simulink model "lineAndEdgeDetection"  (R2018a)
settings: Solver=FixedStepAuto  StartTime=0.0  StopTime=10.0  FixedStep=0.1  RelTol=1e-3
model workspace (MAT data in the model file):
  clusterProximityThreshold = 0.05
  lineTrackingThreshold = 0.2
  netAngleThreshold = 0.314159265359
  scalerho = 0.002
undefined symbols (not defined in the file or in its folder): gray
libraries: visiontextngfix x3, visiontransforms x3, dspindex x2, visionanalysis x1, visionstatistics x1, visiongeotforms x1
settings Model: Creator=vuwij  LastModifiedBy=vuwij
settings DataIOCC: SaveOutput=off  SaveTime=off
settings OptimizationCC: EnhancedBackFolding=on  PassReuseOutputArgsAs=Individual arguments  MaxStackSize=64  OptimizeBlockOrder=speed  DifferentSizesBufferReuse=on  OptimizationCustomize=off
settings DebuggingCC: ParameterTunabilityLossMsg=error
settings HardwareCC: ProdBitPerPointer=32  ProdBitPerSizeT=32  ProdBitPerPtrDiffT=32  ProdLargestAtomicFloat=None  ProdIntDivRoundTo=Undefined  ProdEndianess=Unspecified  ProdWordSize=32  ProdHWDeviceType=Generic->Unspecified (assume 32-bit Generic)
settings SFSimCC: MATLABDynamicMemAlloc=off
settings RTWCC: SystemTargetFile=ert.tlc  HardwareBoard=Robot Operating System (ROS)  TLCOptions="-aInlineSetEventsForThisBaseRateFcn=TLC_FALSE -aSuppressMultiTaskScheduler=TLC_FALSE  -aRateBasedStepFcn=0"  TemplateMakefile=ert_default_tmf  GenerateReport=on  Toolchain=Catkin  IncludeHyperlinkInReport=on  LaunchReport=on  TargetLang=C++  GenerateTraceInfo=on  GenerateTraceReport=on  GenerateTraceReportSl=on  GenerateTraceReportSf=on  GenerateTraceReportEml=on
settings CodeAppCC: ForceParamTrailComments=on  IgnoreCustomStorageClasses=off  OperatorAnnotations=on  SimulinkDataObjDesc=on  SFDataObjDesc=on  InsertBlockDesc=on
settings ERTTargetCC: SupportVariableSizeSignals=on

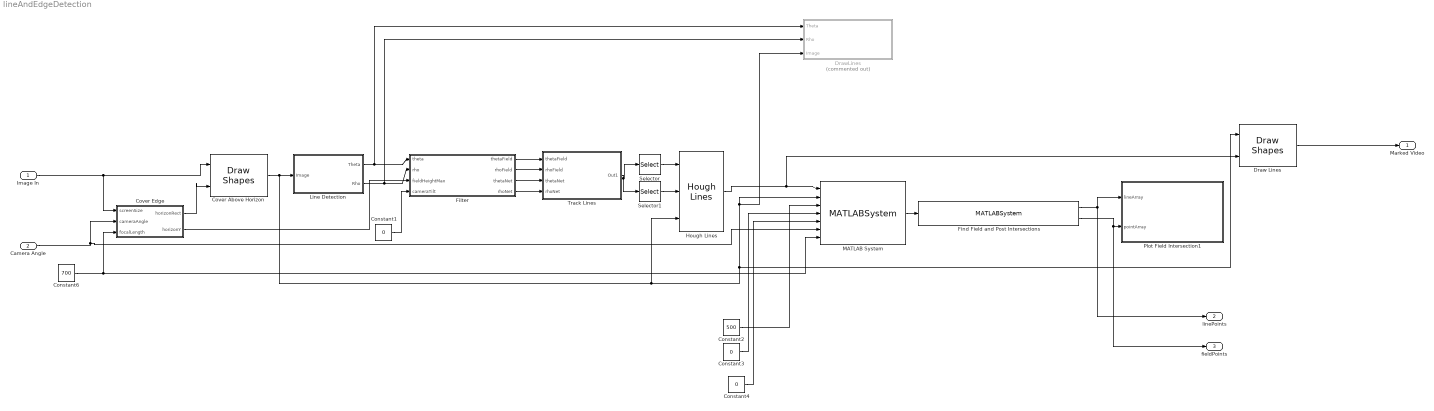
== system lineAndEdgeDetection ==
  Image In : Inport  OutDataTypeStr=uint8  PortDimensions=[480 640]  SampleTime=[0.1,0]
  Camera Angle : Inport  Port=2  PortDimensions=1
  Constant1 : Constant  Value=0
  Constant2 : Constant  Value=500
  Constant3 : Constant  Value=0
  Constant4 : Constant  Value=0
  Constant6 : Constant  Value=700
  Cover Above Horizon : visiontextngfix/Draw Shapes  shape=Rectangles  fill=on  lineWidth=1  fillClrSource=Specify via dialog  display=Black  intensity=200  color=[255 0 0]  opacity=0.8  viewport=Entire image  antialiasing=off  inType=Obsolete  imagePorts=One multidimensional signal  prodOutputMode=Binary point scaling  prodOutputWordLength=32  prodOutputFracLength=14  memoryMode=Specify word length  memoryWordLength=16  memoryFracLength=14  roundingMode=Floor  overflowMode=off
      settings: SourceProductName=Computer Vision System Toolbox
  Cover Edge : MATLAB Function  TreatAsAtomicUnit=on
  Draw Lines : visiontextngfix/Draw Shapes  shape=Lines  fill=off  lineWidth=1  fillClrSource=Specify via dialog  display=White  intensity=200  color=[255 0 0]  opacity=0.6  viewport=Entire image  antialiasing=on  inType=Obsolete  imagePorts=One multidimensional signal  prodOutputMode=Binary point scaling  prodOutputWordLength=32  prodOutputFracLength=14  memoryMode=Specify word length  memoryWordLength=16  memoryFracLength=14  roundingMode=Floor  overflowMode=off
      settings: SourceProductName=Computer Vision System Toolbox
  DrawLines : Subsystem  Commented=on
  Filter : MATLAB Function  TreatAsAtomicUnit=on
  Find Field and Post Intersections : MATLABSystem  System=findFieldAndPostIntersections  SimulateUsing=Interpreted execution
      mask Type: findFieldAndPostIntersections
      mask Display:
      | disp('findFieldAndPostIntersections');
      | port_label('input',1,'lineArray');
      | port_label('output',1,'lineArray');
      | port_label('output',2,'pointArray');
  Hough Lines : visiontransforms/Hough Lines  sineCompMethod=Trigonometric function  thetaRes=pi/180  firstCoeffMode=Specify word length  firstCoeffWordLength=16  firstCoeffFracLength=15  prodOutputMode=Binary point scaling  prodOutputWordLength=32  prodOutputFracLength=16  roundingMode=Nearest  overflowMode=on
      settings: SourceProductName=Computer Vision System Toolbox  SourceProductBaseCode=VP
  Line Detection : Subsystem
  MATLAB System : MATLABSystem  System=map2Dto3D  SimulateUsing=Interpreted execution
      mask Type: map2Dto3D
      mask Display:
      | disp('map2Dto3D');
      | port_label('input',1,'lines');
      | port_label('input',2,'img');
      | port_label('input',3,'robotHeight');
      | port_label('input',4,'d');
      | port_label('input',5,'robotAngle');
      | port_label('input',6,'cameraAngle');
      | port_label('input',7,'focalLength');
      | port_label('output',1,'lines3D');
  Plot Field Intersection1 : MATLAB Function  TreatAsAtomicUnit=on
  Selector : Selector  NumberOfDimensions=2  InputPortWidth=3  IndexOptions=Select all,Index vector (dialog)  Indices=[1 3],1  OutputSizes=1,1
  Selector1 : Selector  NumberOfDimensions=2  InputPortWidth=3  IndexOptions=Select all,Index vector (dialog)  Indices=[1 3],2  OutputSizes=1,1
  Track Lines : Subsystem
  Marked Video : Outport  OutDataTypeStr=uint8  SampleTime=[0,1]
  linePoints : Outport  Port=2  OutDataTypeStr=double  SampleTime=[0,1]
  fieldPoints : Outport  Port=3  OutDataTypeStr=double  SampleTime=[0,1]
  wires:
  Line Detection/1(Theta) -> Filter/1(theta), DrawLines/1(Theta)
  Line Detection/2(Rho) -> Filter/2(rho), DrawLines/2(Rho)
  Constant1/1 -> Filter/4(cameraTilt)
  Filter/2(rhoField) -> Track Lines/2("rhoField ")
  Filter/3(thetaNet) -> Track Lines/3(thetaNet)
  Filter/4(rhoNet) -> Track Lines/4(rhoNet)
  Hough Lines/1 -> MATLAB System/1, Draw Lines/2
  Constant2/1 -> MATLAB System/3
  Constant3/1 -> MATLAB System/4
  Constant4/1 -> MATLAB System/5
  Constant6/1 -> Cover Edge/3(focalLength), MATLAB System/7
  Track Lines/1(Out1) -> Selector/1, Selector1/1
  Selector/1 -> Hough Lines/1
  Selector1/1 -> Hough Lines/2
  Draw Lines/1 -> Marked Video/1
  Cover Above Horizon/1 -> Draw Lines/1, DrawLines/3(Image), MATLAB System/2, Hough Lines/3, Line Detection/1(Image)
  Camera Angle/1 -> Cover Edge/2(cameraAngle), MATLAB System/6
  Cover Edge/1(horizonRect) -> Cover Above Horizon/2
  Filter/1(thetaField) -> Track Lines/1(thetaField)
  Cover Edge/2(horizonY) -> Filter/3(fieldHeightMax)
  Find Field and Post Intersections/2 -> fieldPoints/1, Plot Field Intersection1/2(pointArray)
  MATLAB System/1 -> Find Field and Post Intersections/1
  Image In/1 -> Cover Edge/1(screenSize), Cover Above Horizon/1
  Find Field and Post Intersections/1 -> linePoints/1, Plot Field Intersection1/1(lineArray)

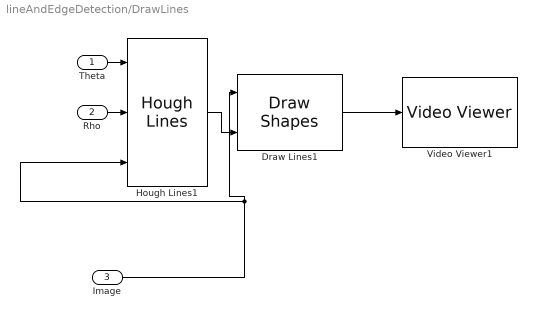
== system lineAndEdgeDetection/DrawLines ==
  Theta : Inport
  Rho : Inport  Port=2
  Image : Inport  Port=3
  Draw Lines1 : visiontextngfix/Draw Shapes  shape=Lines  fill=off  lineWidth=1  fillClrSource=Specify via dialog  display=White  intensity=200  color=[255 0 0]  opacity=0.6  viewport=Entire image  antialiasing=off  inType=Obsolete  imagePorts=One multidimensional signal  prodOutputMode=Binary point scaling  prodOutputWordLength=32  prodOutputFracLength=14  memoryMode=Specify word length  memoryWordLength=16  memoryFracLength=14  roundingMode=Floor  overflowMode=off
      settings: SourceProductName=Computer Vision System Toolbox
  Hough Lines1 : visiontransforms/Hough Lines  sineCompMethod=Trigonometric function  thetaRes=pi/180  firstCoeffMode=Specify word length  firstCoeffWordLength=16  firstCoeffFracLength=15  prodOutputMode=Binary point scaling  prodOutputWordLength=32  prodOutputFracLength=16  roundingMode=Nearest  overflowMode=on
      settings: SourceProductName=Computer Vision System Toolbox  SourceProductBaseCode=VP
  Video Viewer1 : VideoViewer  colormapValue=gray(256)  FigPos=[-205.666666666667 996 1136 624]
  wires:
  Theta/1 -> Hough Lines1/1
  Draw Lines1/1 -> Video Viewer1/1
  Hough Lines1/1 -> Draw Lines1/2
  Image/1 -> Hough Lines1/3, Draw Lines1/1
  Rho/1 -> Hough Lines1/2

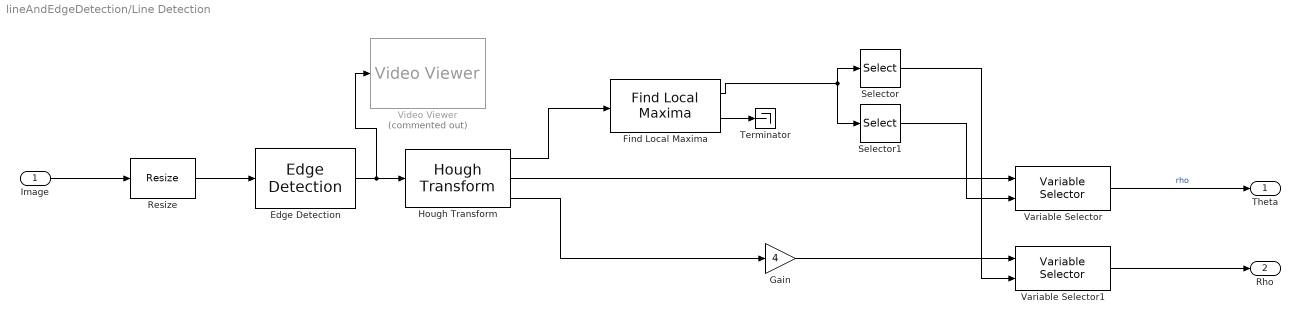
== system lineAndEdgeDetection/Line Detection ==
  Image : Inport
  Edge Detection : visionanalysis/Edge Detection  method=Prewitt  outputType=Binary image  userDefinedThreshold=off  thresholdSource=Input port  threshold=20  thresholdTuning=6  edgeThinning=on  threshold_canny=[0.25 0.60]  autoPercent=70  sigma=1  roundingMode=Floor  overflowMode=off  prodOutputMode=Binary point scaling  prodOutputWordLength=32  prodOutputFracLength=8  prodOutputSlope=2^-8  accumSlope=2^-8  outputSlope=2^-4
      settings: SourceProductName=Computer Vision System Toolbox  SourceProductBaseCode=VP
  Find Local Maxima : visionstatistics/Find Local Maxima  num_peaks=20  nhood_size=[201 51]  src_thresh=Obsolete9b  src_thresh_inuse=Specify via dialog  threshold=27  inputIsHough=on  dt_peak=uint32  isOutVarDim=off  dt_count=uint32
      settings: SourceProductName=Computer Vision System Toolbox  SourceProductBaseCode=VP
  Gain : Gain  Gain=4
  Hough Transform : visiontransforms/Hough Transform  theta_res=pi/180  rho_res=1  out_theta_rho=on  outdtmode=double  firstCoeffMode=Binary point scaling  firstCoeffWordLength=16  firstCoeffFracLength=14  secondCoeffMode=Binary point scaling  secondCoeffWordLength=32  secondCoeffFracLength=16  outputMode=Binary point scaling  outputWordLength=16  outputFracLength=0  accumMode=Binary point scaling  accumWordLength=32  accumFracLength=20  prodOutputMode=Binary point scaling  prodOutputWordLength=32  prodOutputFracLength=20  memoryMode=Binary point scaling  memoryWordLength=32  memoryFracLength=16  roundingMode=Nearest  overflowMode=on
      settings: SourceProductName=Computer Vision System Toolbox  SourceProductBaseCode=VP
  Resize : visiongeotforms/Resize  specify=Output size as a percentage of input size  rfactor=[25 25]  outCols=25  outRows=25  outRowsCols=[25 35]  interp_method=Bilinear  antialias=off  useROI=off  roiFlag=off  prodOutputMode=Binary point scaling  prodOutputWordLength=32  prodOutputFracLength=10  roundingMode=Nearest  overflowMode=on
      settings: SourceProductName=Computer Vision System Toolbox  SourceProductBaseCode=VP
  Selector : Selector  NumberOfDimensions=2  InputPortWidth=2  IndexOptions=Select all,Index vector (dialog)  Indices=1,2  OutputSizes=1,1
  Selector1 : Selector  NumberOfDimensions=2  InputPortWidth=2  IndexOptions=Select all,Index vector (dialog)  Indices=0,1  OutputSizes=1,1
  Terminator : Terminator
  Variable Selector : dspindex/Variable Selector  NumInputs=1  rowsOrCols=Columns  IdxMode=Variable  Elements=[1 3]  ZerOneIdxMode=One-based  errmode=Clip Index  FillMode=on  FillValues=0
  Variable Selector1 : dspindex/Variable Selector  NumInputs=1  rowsOrCols=Columns  IdxMode=Variable  Elements=[1 3]  ZerOneIdxMode=One-based  errmode=Clip Index  FillMode=on  FillValues=0
  Video Viewer : VideoViewer  Commented=on  FigPos=[727 756 635 435]
  Theta : Outport
  Rho : Outport  Port=2
  wires:
  Image/1 -> Resize/1
  Gain/1 -> Variable Selector1/1
  Resize/1 -> Edge Detection/1
  Edge Detection/1 -> Hough Transform/1, Video Viewer/1
  Variable Selector1/1 -> Rho/1
  Variable Selector/1 -> Theta/1  "rho"
  Hough Transform/3 -> Gain/1
  Selector1/1 -> Variable Selector/2
  Selector/1 -> Variable Selector1/2
  Find Local Maxima/1 -> Selector/1, Selector1/1
  Hough Transform/2 -> Variable Selector/1
  Hough Transform/1 -> Find Local Maxima/1
  Find Local Maxima/2 -> Terminator/1

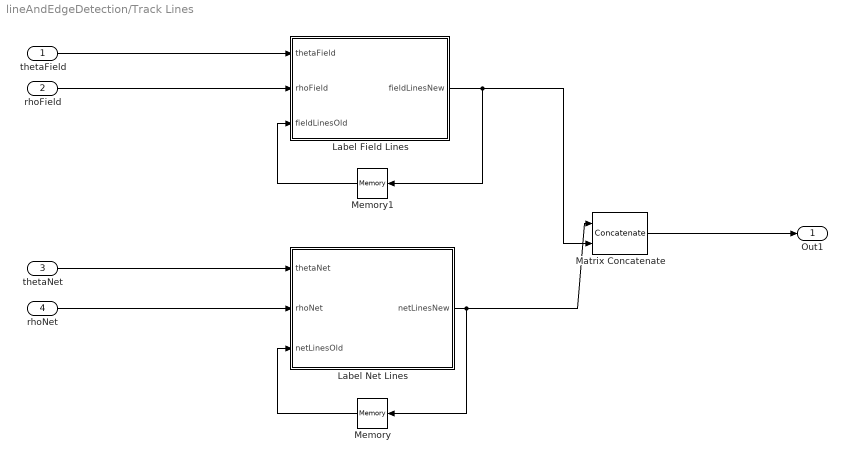
== system lineAndEdgeDetection/Track Lines ==
  thetaField : Inport
  "rhoField " : Inport  Port=2
  thetaNet : Inport  Port=3
  rhoNet : Inport  Port=4
  Label Field Lines : MATLAB Function  TreatAsAtomicUnit=on
  Label Net Lines : MATLAB Function  TreatAsAtomicUnit=on
  Matrix Concatenate : Concatenate  Mode=Multidimensional array
  Memory : Memory  InitialCondition=[0,0;0,0;0,0;0,0]
  Memory1 : Memory  InitialCondition=[0,0;0,0;0,0;0,0;0,0]
  Out1 : Outport
  wires:
  Matrix Concatenate/1 -> Out1/1
  Label Field Lines/1(fieldLinesNew) -> Memory1/1, Matrix Concatenate/2
  Memory1/1 -> Label Field Lines/3(fieldLinesOld)
  thetaField/1 -> Label Field Lines/1(thetaField)
  "rhoField "/1 -> Label Field Lines/2(rhoField)
  Memory/1 -> Label Net Lines/3(netLinesOld)
  Label Net Lines/1(netLinesNew) -> Memory/1, Matrix Concatenate/1
  rhoNet/1 -> Label Net Lines/2(rhoNet)
  thetaNet/1 -> Label Net Lines/1(thetaNet)

== matlab function lineAndEdgeDetection/Cover Edge ==
  data: horizonRect output; horizonY output; screenSize input; cameraAngle input; focalLength input
function [horizonRect, horizonY] = fcn(screenSize, cameraAngle, focalLength)
    [l, w] = size(screenSize);
    
    horizonY = l/2 - tan(cameraAngle) * focalLength;
    horizonRect = uint32([0, 0, w, horizonY]);

== matlab function lineAndEdgeDetection/Track Lines/Label Net Lines ==
  data: thetaNet input; netLinesNew output; rhoNet input; netLinesOld input; lineTrackingThreshold parameter; scalerho parameter
function netLinesNew = labelNetLines(thetaNet, rhoNet, netLinesOld, lineTrackingThreshold, scalerho)
    % Keep the memory of the new lines
    netLinesNew = zeros(4,2);
    if any(netLinesOld)
        netLinesNew = netLinesOld;
    end
    
    % Update if anything changed
    totalLineCount = 0;
    for i = 1:6
       if (thetaNet(i) == 0 && rhoNet(i) == 0)
           continue;
       else
           totalLineCount = totalLineCount + 1;
       end
    end
    
    if (totalLineCount == 2)
        if(rhoNet(2) < rhoNet(1))
            netLinesNew(1,1) = thetaNet(1);
            netLinesNew(1,2) = rhoNet(1);
            netLinesNew(2,1) = thetaNet(2);
            netLinesNew(2,2) = rhoNet(2);
        else
            netLinesNew(1,1) = thetaNet(2);
            netLinesNew(1,2) = rhoNet(2);
            netLinesNew(2,1) = thetaNet(1);
            netLinesNew(2,2) = rhoNet(1);
        end
    end
    
    if (totalLineCount == 1)
        if(netLinesNew(1,1) ~= 0 && netLinesNew(2,1) ~= 0 && netLinesNew(1,2) ~= 0 && netLinesNew(2,2) ~= 0) % Seen both lines already
            theta1 = netLinesNew(1,1);
            rho1 = netLinesNew(1,2) * scalerho;
            theta2 = netLinesNew(2,1);
            rho2 = netLinesNew(2,2) * scalerho;
            
            thetaNew = thetaNet(1);
            rhoNew = rhoNet(1) * scalerho;
            
            distLeftLine = norm([thetaNew - theta1, rhoNew - rho1]);
            distRightLine = norm([thetaNew - theta2, rhoNew - rho2]);
            
            if distLeftLine < distRightLine
%                 netLinesNew(2,1) = netLinesNew(2,1) + thetaNet(1) - netLinesNew(1,1);
%                 netLinesNew(2,2) = netLinesNew(2,2) + rhoNet(1) - netLinesNew(1,2);
%                 
                netLinesNew(1,1) = thetaNet(1);
                netLinesNew(1,2) = rhoNet(1);
            else
%                 netLinesNew(1,1) = netLinesNew(1,1) + thetaNet(1) - netLinesNew(2,1);
%                 netLinesNew(1,2) = netLinesNew(1,2) + rhoNet(1) - netLinesNew(2,2);
%                 
                netLinesNew(2,1) = thetaNet(1);
                netLinesNew(2,2) = rhoNet(1);
            end
        else
            netLinesNew(1,1) = thetaNet(1);
            netLinesNew(1,2) = rhoNet(1);
        end
    end
end

== matlab function lineAndEdgeDetection/Filter ==
  data: thetaField output; theta input; rhoField output; rho input; thetaNet output; rhoNet output; fieldHeightMax input; cameraTilt input; scalerho parameter; clusterProximityThreshold parameter; netAngleThreshold parameter
function [thetaField, rhoField, thetaNet, rhoNet]  = filterLines(theta, rho, fieldHeightMax, cameraTilt, scalerho, clusterProximityThreshold, netAngleThreshold)
    % Fix the negative lines
    lines = [transpose(theta),transpose(rho) * scalerho];
    for i = 1:length(lines)
       if lines(i,2) < 0
          lines(i,1) = lines(i,1) + pi;
          lines(i,2) = -lines(i,2);
       end
       if lines(i,1) > pi
          lines(i,1) = lines(i,1) - 2 * pi; 
       end
    end
    
    sumdbest = 1000000;
    kbest = 0;
    linesFilteredBest = 0;
        
    % Proper clustering
    for k = 3:6
        [~,C,sumd] = kmeans(lines,k,'Replicates',1,'MaxIter',15);
        tooclose = 0;
        for i = 1:k
            for j = 1:k
                if i <= j 
                    continue;
                end
                if(norm(C(i,:)-C(j,:)) < clusterProximityThreshold)
                    tooclose = 1;
                end
            end
        end
        
        if(tooclose == 1)
            continue
        end
        
        if (mean(sumd) < sumdbest)
            sumdbest = mean(sumd);
            kbest = k;
            linesFilteredBest = C;
        end
    end
   

    
    % Plot the data
%     plot(lines(:,1),lines(:,2), 'o')
%     hold on;
%     plot(linesFilteredBest(:,1),linesFilteredBest(:,2), 'x')
%     title 'Rho and theta data data for lines'
%     xlabel 'Theta'
%     ylabel 'Rho'
%     xlim([-pi pi])
%     ylim([0 640 * scalerho])
%     grid minor
%     hold off;
    
    % Figure out which is part of the field
    thetaField = zeros(1,6);
    rhoField = zeros(1,6);
    thetaNet = zeros(1,6);
    rhoNet = zeros(1,6);
    fieldLineCount = 0;
    netLineCount = 0;
    
    for i = 1:kbest
        if (linesFilteredBest(i,1) < netAngleThreshold + cameraTilt && linesFilteredBest(i,1) > -netAngleThreshold + cameraTilt)
            netLineCount = netLineCount + 1;
            thetaNet(netLineCount) = transpose(linesFilteredBest(i,1));
            rhoNet(netLineCount) = transpose(linesFilteredBest(i,2)) / scalerho;
        else
            %Todo fix this so thresholding properly
           if linesFilteredBest(i,2) > fieldHeightMax * scalerho || (linesFilteredBest(i,1) < 0 && linesFilteredBest(i,1) > - pi/3)
               fieldLineCount = fieldLineCount + 1;
               thetaField(fieldLineCount) = transpose(linesFilteredBest(i,1));
               rhoField(fieldLineCount) = transpose(linesFilteredBest(i,2)) / scalerho;
           end
        end
    end  
end

== matlab function lineAndEdgeDetection/Track Lines/Label Field Lines ==
  data: thetaField input; fieldLinesNew output; rhoField input; fieldLinesOld input; lineTrackingThreshold parameter; scalerho parameter
function fieldLinesNew = labelFieldLines(thetaField, rhoField, fieldLinesOld, lineTrackingThreshold, scalerho)
    % Keep the memory of the new lines
    % Line 1 - Enemy Back Line
    % Line 2 - Left Line
    % Line 3 - Right Line
    % Line 4 - Friendly Back Line
    % Line 5 - Center Line
    fieldLinesNew = zeros(5,2);

    if any(fieldLinesOld)
        fieldLinesNew = fieldLinesOld;
    end
    
    % Sort all the lines by theta
    [thetaFieldSorted, I] = sort(thetaField(1:5));
    rhoFieldSorted = rhoField(I);
    
    fieldLinesNew(1:5,1) = thetaFieldSorted(1:5);
    fieldLinesNew(1:5,2) = rhoFieldSorted(1:5);
    
%     if ~any(fieldLinesNew(1:5,1:2))
%         fieldLinesNew(1:5,1) = thetaFieldSorted(1:5);
%         fieldLinesNew(1:5,2) = rhoFieldSorted(1:5);
%     else
%         % If any of the line are close to the lines then assign them to new
%         % location, then assign second closest line to another line, then
%         % assign 3rd closest, then 2nd then 1st
%         iset = 1:5;
%         jset = 1:5;
%         
%         for c = 1:5
%             mindist = 100000;
%             imin = 1;
%             jmin = 1;
%             
%             for i = iset
%                 for j = jset
%                     if (i == 0 || j == 0)
%                         continue; 
%                     end
%                     
%                     dist = norm([thetaFieldSorted(j) - fieldLinesNew(i,1), rhoFieldSorted(j) * scalerho - fieldLinesNew(i,2) * scalerho]);
%                     if dist < mindist
%                         mindist = dist;
%                         imin = i;
%                         jmin = j;
%                     end
%                 end
%             end
%             
%             iset(imin) = 0;
%             jset(jmin) = 0;
%             
%             if(mindist < lineTrackingThreshold)
%                 fieldLinesNew(imin,1) = thetaFieldSorted(jmin);
%                 fieldLinesNew(imin,2) = rhoFieldSorted(jmin);
%             end
%         end
%     end
end

== matlab function lineAndEdgeDetection/Plot Field Intersection1 ==
  data: lineArray input; pointArray input
function plotPointArray(lineArray, pointArray)
    drawfield(lineArray(5:9,[1,2,4,5]), pointArray);
